simulink model "thruster_model"  (R2025b)
settings: Solver=FixedStepAuto  StartTime=0.0  StopTime=tspan  FixedStep=dt  RelTol=1e-3
undefined symbols (not defined in the file): bs, Imech, kf0, kf1, kT, kT0, kv, Qhyd0, w0
settings Model: Creator=rubystanton  LastModifiedBy=rubystanton
settings DataIOCC: ExternalInput=inputStructure  LoadExternalInput=on

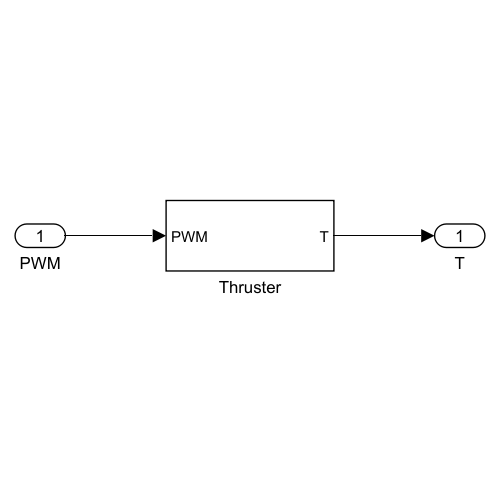
[thumbnail: Simulink's stored preview of the top-level diagram]
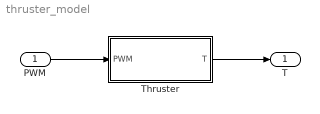
== system thruster_model ==
  PWM : Inport
  Thruster : Subsystem
  T : Outport
  wires:
  Thruster/1(T) -> T/1
  PWM/1 -> Thruster/1(PWM)

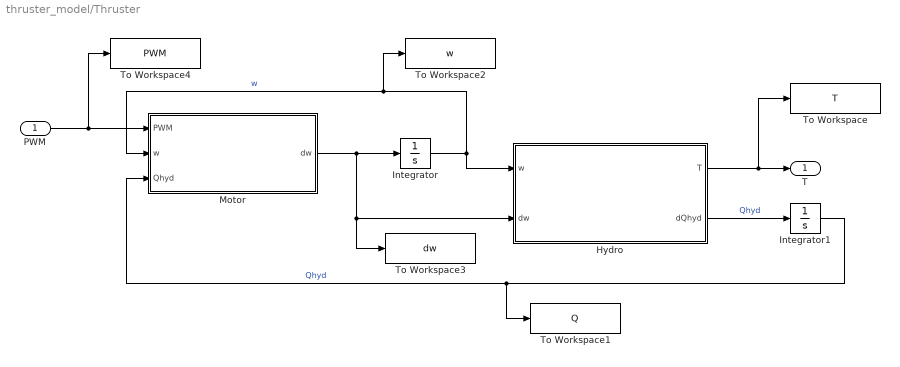
== system thruster_model/Thruster ==
  PWM : Inport
  Hydro : MATLAB Function  TreatAsAtomicUnit=on
  Integrator : Integrator  InitialCondition=w0
  Integrator1 : Integrator  InitialCondition=Qhyd0
  Motor : MATLAB Function  TreatAsAtomicUnit=on
  To Workspace : ToWorkspace  VariableName=T  SaveFormat=Timeseries  SampleTime=-1
  To Workspace1 : ToWorkspace  VariableName=Q  SaveFormat=Timeseries  SampleTime=-1
  To Workspace2 : ToWorkspace  VariableName=w  SaveFormat=Timeseries  SampleTime=-1
  To Workspace3 : ToWorkspace  VariableName=dw  SaveFormat=Timeseries  SampleTime=-1
  To Workspace4 : ToWorkspace  VariableName=PWM  SaveFormat=Timeseries  SampleTime=-1
  T : Outport
  wires:
  PWM/1 -> To Workspace4/1, Motor/1(PWM)
  Motor/1(dw) -> To Workspace3/1, Hydro/2(dw), Integrator/1
  Integrator/1 -> To Workspace2/1, Motor/2(w), Hydro/1(w)  "w"
  Hydro/1(T) -> To Workspace/1, T/1
  Hydro/2(dQhyd) -> Integrator1/1  "Qhyd"
  Integrator1/1 -> Motor/3(Qhyd), To Workspace1/1  "Qhyd"

== matlab function thruster_model/Thruster/Hydro ==
  data: T output; w input; dQhyd output; dw input; kT0 parameter; kT parameter; Imech parameter; bs parameter
function [T,dQhyd] = HydroModel(w,dw, kT0, kT, Imech,bs)
    dQhyd = bs*dw; %Brachmeyer et al (2000) + i need a break
    T = kT0*w + kT*w^2; %Aras et al model (2013)
end

== matlab function thruster_model/Thruster/Motor ==
  data: PWM input; w input; dw output; Qhyd input; kf1 parameter; kf0 parameter; kv parameter
function dw  = DCBrushlessModel(PWM,w,Qhyd,kf1, kf0, kv)
    V = 14.8; %[V]
    f = 24e6; %[Hz]
    Vrms = V*sqrt(PWM*f); % Average Voltage
    if(PWM<1530 && PWM>1470)
        dw=0; %from T-200 table
    else
        friction = kf1*w + kf0*2/pi*atan(20*w); %Brachmeyer 2000
        dw = kv*Vrms - friction - Qhyd; %Brachmeyer 2000
    end
end
